simulink model "Integration2022b_May06"  (R2022b)
settings: Solver=FixedStepAuto  StartTime=0.0  StopTime=inf  RelTol=1e-3
model workspace (MAT data in the model file):
  L = 4.165
  SL_ROS_VariableLengthArrays_MaxSizes : object (value not decoded)
  finalint = 0
  firstWarning = 1
  originalScenarioChecksum = '114339432DE22364D47BB28FC96DC10C'
values from neighbouring files (symbols this model uses):
  D = cross(B-A,C-A)    [HelperCalculateEgoRefPathInfo.m]
  data =     [Part_of_MCity.mat]    (also in curvedroad_Bhanu.mat; plotWPScript.m = [data, [out.x.Data(:, :, i); out.y.Data(:, :, i)]])
  x = [Vertices(Na,1) Vertices(:,1) Vertices(Nb,1)]    [HelperCalculateEgoRefPathInfo.m]    (also in HelperConvertDSPoseToSim3D.m = actor(1).Position(1); xpts.mat = [-29.9023190589 -34.2715935353 -19.4160603154 -19.4160603154)
  y = [Vertices(Na,2) Vertices(:,2) Vertices(Nb,2)]    [HelperCalculateEgoRefPathInfo.m]    (also in HelperConvertDSPoseToSim3D.m = actor(1).Position(2); VehicleOutputFcn.m = [x(1);x(2); x(3); x(4); x(5);x(6)]; ypts.mat = [-62.3254015256 -62.9079714558 -51.8391427821 -48.6350081661)
  z = zeros(1, length(interpX))    [HelperCalculateEgoRefPathInfo.m]
undefined symbols (not defined in the file or in its folder): MinVelocity, WB
libraries: ros2lib x13, mpcsigdimcheck_private x10, robotalgslib x1, mpclib x1, drivingvehiclecontroller x1, slpidlib x1
(part 4 of 5)

== matlab function Integration2022b_May06/Environment // SF Detections ==
  data: matrixA input; objectAhead output; mostImpObjectPose output; objectRelativeVelocity output; objectDistance output; railroadGate output; sceneId output; noLight output; red output; yellow output; green output; trafficSignalType output; trafficSignType output; egoLane output; minRelativeVelocity output; minRelativeDistance output; nextRoadSpeed output; roadSpeed output; leftLaneMarkInfo output; rightLaneMarkInfo output; laneNumber output; LatDistanceToScene output; LongDistanceToScene output; matrixB input; matrixC input; matrixD input; matrixE input; matrixF input; transitionFlag input; roadSpeed input; defaultRoadSpeed input; SDist input; CurrentPose input; signX output; signY output
function [objectAhead, mostImpObjectPose, objectRelativeVelocity, objectDistance, railroadGate, sceneId,...
            noLight, red, yellow, green, trafficSignalType, trafficSignType, egoLane, minRelativeVelocity, minRelativeDistance, nextRoadSpeed, roadSpeed, ...
            leftLaneMarkInfo, rightLaneMarkInfo, laneNumber, LatDistanceToScene, LongDistanceToScene, signX, signY] = ...
            PerceptionData(matrixA, matrixB, matrixC, matrixD, matrixE, matrixF, transitionFlag, roadSpeed, ...
            defaultRoadSpeed, SDist, CurrentPose)
 
    % Get sizes of matrices
    sizeA = size(matrixA);                              % Object detections, 
    sizeB = size(matrixB);                              % Traffic signals,
    sizeC = size(matrixC);                              % Traffic signs
    sizeD = size(matrixD);                              % Road state
    sizeE = size(matrixE);                              % Limit line
    sizeF = size(matrixF);                              % Lane markings
    offsetToFront = 2.1336;                             % Offset to the front of the vehicle, from the driver's seat
    % lengthOfCar = 4.1656;                             % Car length
    % Initialization: relevant to matrix A
    objectAhead = 0;                                    % Boolean
    railroadGate = 0;                                   % Boolean
    mostImpObjectPose = zeros(2, 1);
    objectDistance = 40;
    objectRelativeVelocity = 0;                         % [changed from 10 to 0]
    sceneId = 0; 

    % Initialization: relevant to matrix B
    noLight = 0;                                        % Boolean
    trafficSignalType = 0;
    red = zeros(1,6);                                   % Encoded as boolean
    green = zeros(1,3);                                 % Encoded as boolean
    yellow = zeros(1,6);                                % Encoded as boolean
    trafficSignalId = 0;
    % Initialization: relevant to matrix C
    trafficSignType = 0;
    LongDistanceToScene = -1;
    LatDistanceToScene = -1;
    nextRoadSpeed = 7;
    LongDistanceToTrafficSign = 40;
    LatDistanceToTrafficSign=10;
   

    LongDistanceToTrafficSignal = 40;
    LatDistanceToTrafficSignal = 10;
    maxIntersectionLength = 32;                         % Dimension of intersection [m]
    % roadSpeed = defaultRoadSpeed;                       % Initialize to default road speed [mph]
    signLatPose=-1;
    signLongPose=-1;
    egoLane = matrixD(1, 4);
    laneNumber = matrixD(1, 9);
    
    % Relative to ego coordinates
    leftLaneIndex = 0;                                  % Index of left lane marking
    rightLaneIndex = 0;                                 % Index of right lane marking
    leftLaneMarkInfo = zeros(1, 2);                     % Color and type of lane marking
    rightLaneMarkInfo = zeros(1, 2);                    % Color and type of lane marking
    distanceToLaneMarking = zeros(1, sizeF(1));
    
    for i = 1:sizeA(1)                                  % Looping over rows of Matrix A (Different Detections)
       objObjectId = matrixA(i, 1);                     % Object ID
       objObjectType = matrixA(i, 2);                   % Object type
       
       if objObjectType == -1
           break;
       end
    
       lateralPose = matrixA(i, 3);                     % Relative lateral (X) Pose
       longitudinalPose = matrixA(i, 4);                % Relative longitudinal (Y) Pose
       relativeLongVelocity = matrixA(i, 5);            % Relative longitudinal velocity
       relativeLateralVelocity = matrixA(i, 6);         % Relative lateral velocity
       relativeLane = matrixA(i, 7);                    % Relative lane
       dynamicProperty = matrixA(i, 8);                 % Dynamic property (static/dynamic)
       objectCourse = head - (90 - matrixA(i, 9));      % heading in IMU frame (North = 0, clockwise shift) converted to vehicle frame
       netRelativeVelocity = sqrt(relativeLongVelocity^2 + relativeLateralVelocity^2);

    % Static obstacles in our lane
        if (dynamicProperty == 1 && relativeLane == 1) || objObjectId == 5 && (longitudinalPose <= SDist)
            statObstacleFlag = 1;
            statObstacleLocation = double([objectLatitude objectLongitude]);
        end
    % Relative Lane Code = 2: opposing, 3: left lane, 4: right lane 
    % Dynamic obstacles detection
        if (objObjectType > 0 && objObjectType <= 3) && (dynamicProperty == 3 || dynamicProperty == 4) % check if moving vehicle
            if relativeLane == 1 && (objectCourse >= CurrentPose(3) - 15 && objectCourse <= CurrentPose(3) + 15) % cushion of 15 degrees +/- ego vehicle heading to detect same direction travel
                dynamicACCFlag = 1;
                objectAhead = 1;
                objectDistance = min(objectDistance, longitudinalPose); % change to lat/long reading
            end

            if relativeLane == 2 && abs(objectCourse) > 160 && abs(objectCourse < 290) % discuss where relative heading angle starts from: car x or car y or keep it local heading only?
                oppVehicleFlag = 1;

            end
            if relativeLane > 2 && relativeLane < 6 && objectCourse >= 90 - 15 && objectCourse < 90 + 15
                vehicleFlag = 1;
            end

    % Pedestrian at Crosswalk
       if objObjectType == 4 && (relativeLane > 1 && relativeLane < 7) && (dynamicProperty == 3 || dynamicProperty == 4) % check if moving pedestrian (lane, moving, pedestrian check)
           pedestrianFlag = 1;
           objectAhead = 1;
           pedestrianDistance = 
           pedestrianVelocity = netRelativeVelocity;
       end

       if longitudinalPose <= objectDistance
          objectRelativeVelocity = relativeLongVelocity;
          % objectTrackedId = objObjectId;
          mostImpObjectPose(1:2, 1) = [lateralPose; longitudinalPose];
       end

          
       
       % railroad gate detected (closed)
       elseif relativeLane == 1 && objObjectType == 7 
           railroadGate = 1;
       end
end

    
    % Checking which traffic sign is important, its type and position
    for i = 1:sizeC(1)
        % if no detection, scene variables should be -1
%         signLateralPose = matrixC(i, 3);
%         signLongitudinalPose = matrixC(i, 4);
        signObjectId = matrixC(i, 1);
        signType = matrixC(i, 2);
        signX = matrixC(i, 6);
        signY = matrixC(i, 7);
        
        
        % distanceToTrafficSign = sqrt(signX^2 + signY^2);
        if signObjectId == -1 % || matrixD(1, 8) == -1
            break;
        else
            % if there's a known sign and it is not a speed limit
            val1 = (signX - CurrentPose(1))*sind(CurrentPose(3));
            val2 = (signY - CurrentPose(2))*cosd(CurrentPose(3));
            val3 = (signX - CurrentPose(1))*cosd(CurrentPose(3));
            val4 = (signY - CurrentPose(2))*sind(CurrentPose(3));
            signLongitudinalPose = (signX - CurrentPose(1))*sind(90 - CurrentPose(3)) + (signY - CurrentPose(2))*cosd(90 - CurrentPose(3));
            signLateralPose = (signX - CurrentPose(1))*cosd(90 - CurrentPose(3)) - (signY - CurrentPose(2))*sind(90 - CurrentPose(3)); % signY - CurrentPose(2);
            
            if signObjectId > 0 && signType > 2
                LongDistanceToTrafficSign = min(LongDistanceToTrafficSign, abs(signLongitudinalPose));

                % most important traffic sign
                if abs(signLongitudinalPose) <= LongDistanceToTrafficSign
                   trafficSignType = signType;
                   
                   LatDistanceToTrafficSign = signLateralPose;
                   LongDistanceToTrafficSign = signLongitudinalPose;
                end

            elseif signObjectId > 0 && (signType > 0 && signType <= 2)
                
                if signType == 1
                    if (matrixD(1, 2) <= roadSpeed) && matrixD(1, 3) < 8             % set velocity-distance linear equation
                        roadSpeed = matrixD(1, 2);
                        nextRoadSpeed = matrixD(1, 2);
                    elseif matrixD(1, 8) ~= 0
                        roadSpeed = matrixD(1, 8);
                        nextRoadSpeed = matrixD(1, 2);
                    else
                        roadSpeed = defaultRoadSpeed;
                        nextRoadSpeed = matrixD(1, 2);
                    end
%                 elseif signType == 2
%                     if matrixD(1, 8) ~= roadSpeed
%                         roadSpeed = matrixD(1, 8) * 0.621;
%                     else
%                         roadSpeed = roadSpeed;
%                     end
                end              
                
            end
        
        end
    end
    
    % Checking which traffic light is important, its colour and position
    for i = 1:sizeD(1)
        
        % No active traffic light detected
        if matrixD(i, 1) == 0
            break;
        else
            % For all traffic light detections
            for j = 1:sizeB(1)
        
                if matrixB(j, 1) == -1
                    break;
                else
                    trafficSignalId = matrixD(i, 1);
                    signalObjectId = matrixB(j, 1);
                    signalHeadType = matrixB(j, 2);
%                     signalLateralPose = matrixB(j, 3);
%                     signalLongitudinalPose = matrixB(j, 4);
                    signalX = matrixB(j, 21);
                    signalY = matrixB(j, 22);
                    signalLongitudinalPose = (signalX - CurrentPose(1))*cosd(90 - CurrentPose(3)) - (signalY - CurrentPose(2))*sind(90 - CurrentPose(3));
                    signalLateralPose = (signalX - CurrentPose(1))*sind(90 - CurrentPose(3)) + (signalY - CurrentPose(2))*cosd(90 - CurrentPose(3));
            
                    % making sure same traffic light is being referred to
                    if trafficSignalId == signalObjectId
            
                        % [solid, flashing, left, flashingLeft, right, flashingRight]
                        red = [matrixB(j, 6), matrixB(j, 9), matrixB(j, 11), matrixB(j, 14), matrixB(j, 16), matrixB(j, 19)];
                        
                        % [solid, flashing, left, flashingLeft, right, flashingRight]
                        yellow = [matrixB(j, 7), matrixB(j, 10), matrixB(j, 12), matrixB(j, 15), matrixB(j, 17), matrixB(j, 20)];
                        
                        % [1:solid, 2:left, 3:right]
                        green = [matrixB(j, 8), matrixB(j,13), matrixB(j, 18)];
                        
                        noLight = matrixB(j, 5);
                        trafficSignalType = signalHeadType;  
                        LongDistanceToTrafficSignal = signalLongitudinalPose;
                        LatDistanceToTrafficSignal = signalLateralPose;
                    end
                end
            end
        end
    end
    
    %{
        if traffic signal distance is less than traffic sign distance
        distance to the limit line is determined here
    %}
    if LongDistanceToTrafficSignal < LongDistanceToTrafficSign
        sceneId = 8;                    % For a Traffic Light
        LongDistanceToScene = LongDistanceToTrafficSignal;
        LatDistanceToScene = LatDistanceToTrafficSignal;
        
        
        for i = 1:sizeE(1)
            if matrixE(i, 1) == -1
                break;
            else   
%                 limitLineLongitudinalPose = matrixE(i, 3);
%                 limitLineLateralPose = matrixE(i, 2);
                
                limitLineX = matrixE(i, 5); 
                limitLineY = matrixE(i, 6);
                limitLineLongitudinalPose = (limitLineX - CurrentPose(1))*sind(90 - CurrentPose(3)) + (limitLineY - CurrentPose(2))*cosd(90 - CurrentPose(3));
                limitLineLateralPose = (limitLineX - CurrentPose(1))*cosd(90 - CurrentPose(3)) - (limitLineY - CurrentPose(2))*sind(90 - CurrentPose(3)); % limitLineY - CurrentPose(2);

                
%                 relDistanceToLimitLine = norm([limitLineLongitudinalPose,limitLineLateralPose]);
                

%                 limitLineLateralPose = CurrentPose(1) + offsetToFront*cosd(CurrentPose(3)) + relDistanceToLimitLine*cosd(atan2d(limitLineLongitudinalPose,limitLineLateralPose));
%                 limitLineLongitudinalPose = CurrentPose(2) + offsetToFront*sind(CurrentPose(3)) + relDistanceToLimitLine*sind(atan2d(limitLineLongitudinalPose,limitLineLateralPose));
                
                % Below: 
                if matrixE(i, 4) == 1
                    LongDistanceToScene = limitLineLongitudinalPose ;
                    LatDistanceToScene = limitLineLateralPose;
                else
                    if matrixE(i, 1) ~= 0
                        LongDistanceToScene = limitLineLongitudinalPose;
                        LatDistanceToScene = limitLineLateralPose;
                    else
                        LongDistanceToScene = LongDistanceToTrafficSignal - maxIntersectionLength; % modify as of April 28!
                        LatDistanceToScene = LatDistanceToTrafficSignal; % Dummy Value: Modify case above. Lateral Distance is Needed.
                    end
                    
                end
            end
        end
    
    elseif LongDistanceToTrafficSignal > LongDistanceToTrafficSign
        for i = 1:sizeE(1)
            if matrixE(i,1) == -1
                break;
            else
                limitLineX = matrixE(i, 5);
                limitLineY = matrixE(i, 6);
                limitLineLongitudinalPose = (limitLineX - CurrentPose(1))*sind(90 - CurrentPose(3)) + (limitLineY - CurrentPose(2))*cosd(90 - CurrentPose(3));
                limitLineLateralPose = (limitLineX - CurrentPose(1))*cosd(90 - CurrentPose(3)) - (limitLineY - CurrentPose(2))*sind(90 - CurrentPose(3)); % limitLineY - CurrentPose(2);

%                 relDistanceToLimitLine = norm([limitLineLongitudinalPose,limitLineLateralPose]);
%                 limitLineLateralPose = 0*CurrentPose(1) + offsetToFront*cosd(CurrentPose(3)) + relDistanceToLimitLine*cosd(atan2d(limitLineLongitudinalPose,limitLineLateralPose));
%                 limitLineLongitudinalPose = 0*CurrentPose(2) + offsetToFront*sind(CurrentPose(3)) + relDistanceToLimitLine*sind(atan2d(limitLineLongitudinalPose,limitLineLateralPose));
                
                if matrixE(i, 4) == 1
                    LongDistanceToScene = limitLineLongitudinalPose;
                    LatDistanceToScene = limitLineLateralPose;
                else
                    LongDistanceToScene = LongDistanceToTrafficSign;
                    LatDistanceToScene = LatDistanceToTrafficSign;
                end
%                 LongDistanceToScene = LongDistanceToTrafficSign;
%                 LatDistanceToScene = LatDistanceToTrafficSign;
            end
        end
        % LongdistanceToScene = LongdistanceToTrafficSign;   
        % LatDistanceToScene = LatDistanceToTrafficSign;
        switch trafficSignType
            case 3
                sceneId = 7;                % Stop sign
            case 4
                sceneId = 6;                % Yield sign
            case 10
                sceneId = 10;               % Railroad crossing
            case 11
                sceneId = 11;               % Crosswalk
        end
    end

    % *****************************
    % develop logic for unknown detections (all matrices - traffic lights,
    % signs, limit lines, objects, lane markings
    % *****************************

    % If the ego is transitioning from one scene to another
    if transitionFlag == 1
        minRelativeVelocity = objectRelativeVelocity;
        minRelativeDistance = objectDistance;
    else
        minRelativeVelocity = objectRelativeVelocity;
        minRelativeDistance = min(LongDistanceToScene, objectDistance);
    end

    % Lane markings using matrixF
%     for i = 1:sizeF(1)
%         if matrixF(i, 1) == -1
%             break;
%         else
%             distanceToLaneMarking(i) = matrixF(i, 2); % check with perception about the values of this variable
%             [~, laneIndexLeft] = max(distanceToLaneMarking(distanceToLaneMarking < 0));
%             [~, laneIndexRight] = min(distanceToLaneMarking(distanceToLaneMarking > 0));
%             leftLaneMarkInfo = matrixF(laneIndexLeft, 3:4);
%             rightLaneMarkInfo = matrixF(laneIndexRight, 3:4);
%         end
%     end
end

== matlab function Integration2022b_May06/SF Dynamic ==
  data: matrixA input; matrixC input; dynamicRelativeVelocity output; CurrentPose input; distance2Scene input; signX input; signY input; egoVelocity input
function dynamicRelativeVelocity   = TrafficSignAssist(matrixA, matrixC, CurrentPose, distance2Scene, signX, signY, egoVelocity)

offsetToFront = 2.1336;                             % Offset to the front of the vehicle, from the driver's seat
lengthOfCar = 4.1656;                               % Car length
% Initialization: relevant to matrix A
objectAhead = 0;                                    % Boolean
railroadGate = 0;                                   % Boolean
mostImpObjectPose = zeros(2, 1);
objectRelativeDistance = 40;
dynamicRelativeVelocity = 0;                         % [changed from 10 to 0]

maxAccel = 2;
timeAcc = sceneSpeed/maxAccel;
dd = 0.5 * maxAccel * (timeAcc^2);
timeConstantVel = (19 - dd) / SceneSpeed;
totalTime = timeAcc + timeConstantVel;
timeSafe = 1; % Adjusted for other conditions (e,g. weather, road condition ...)
timeOfArrivalThreshold = totalTime + timeSafe;
vehicleClear2GoFlag = 0;

egoSSPriority = 1;
ToAClearance = 1;
ActorHeading = zeros(4,1);
actorExitang = zeros(4,1);

% tempPriority = zeros(numCars+1,1);
d = zeros(10, 5); % distance, velocity, time, location (wrt ego), exit (leaving ints)
Objang = zeros(10, 1);
% priorityTable = zeros(numCars+1, 5);
egoExitang = egoPose(3) - atan2d(midpoint(2)-egoPose(2),midpoint(1)-egoPose(1)); % 0 deg = straight , + = right
egoExitdist = sqrt((midpoint(2)-egoPose(2))^2+(midpoint(1)-egoPose(1))^2);



%%%%%%%%%%%%%%%%%%
intersectionOffset = 15;
timeOfArrival = 1e3;


for i = 1:sizeA(1)                                  % Looping over rows of Matrix A (Different Detections)
   objObjectId = matrixA(i, 1);                     % Object ID
   objObjectType = matrixA(i, 2);                   % Object type
   
   if objObjectType == -1
       break;
   end


   lateralPose = matrixA(i, 3);                     % Relative lateral (X) pose
   longitudinalPose = matrixA(i, 4);                % Relative longitudinal (Y) pose

   relativeLongVelocity = matrixA(i, 5);            % Relative longitudinal velocity
   relativeLateralVelocity = matrixA(i, 6);         % Relative lateral velocity

   relativeLane = matrixA(i, 7);                    % Relative lane
   dynamicProperty = matrixA(i, 8);                 % Dynamic property (static/dynamic)

   objectX = matrixA(i, 10);                        % Object X
   objectY = matrixA(i, 11);                        % Object Y

   objectCourse = matrixA(i, 9));                   % heading in IMU frame converted to vehicle frame

   objectHeading = 90 - objectCourse;
   if objectHeading < -180
       objectHeading = objectHeading + 360;
   elseif abs(objectHeading) == 180
       objectHeading = abs(objectHeading);
   end

   netRelativeVelocity = sqrt(relativeLongVelocity^2 + relativeLateralVelocity^2);


% Relative Lane Code = 2: opposing, 3: left lane, 4: right lane

% Dynamic obstacles detection
    if (objObjectType > 0 && objObjectType <= 3) && (dynamicProperty == 2 || dynamicProperty == 3 && dynamicProperty == 4) % check if moving vehicle
        % First if condition: ACC flag
        if relativeLane == 1 && longitudinalPose <= objectRelativeDistance && (objectCourse >= CurrentPose(3) - 15 && objectCourse <= CurrentPose(3) + 15) % cushion of 15 degrees +/- ego vehicle heading to detect same direction travel
            dynamicACCFlag = 1;
            objectRelativeDistance = longitudinalPose;
            if relativeLongVelocity < 0
                dynamicRelativeVelocity = -netRelativeVelocity;
            else
                dynamicRelativeVelocity = netRelativeVelocity;         % net relative velocity if velocity >= 0
            end
            
        end
        

        % Second if condition: Incoming vehicle (clear 2 go) flag
        offsetAngle = CurrentPose(3) + 45;

        if offsetAngle > 180
            offsetAngle = (offsetAngle - 360);

        intersectionMidpt = [signX + intersectionOffset*cosd(offsetAngle); signY + intersectionOffset*sind(offsetAngle)];
        % incoming vehicles to midpoint

        incomingAngle = atan2d(intersectionMidpt(2) - objectY, intersectionMidpt(1) - objectX);
        objDistanceMidpt = norm(intersectionMidpt - [objectX; objectY]); % distance from incoming ehicle to intersection midpt
        % if objDistanceMidpt > 1e4
        %     objDistanceMidpt = 100;

        velocityXY = [cosd(90 - CurrentPose(3)) -sind(90 - CurrentPose(3)); sind(90 - CurrentPose(3)) cosd(90 - CurrentPose(3))]' * [relativeLateralVelocity; relativeLongVelocity];


        if velocityXY > 0.05
            timeOfArrival = min(timeOfArrival, objDistanceMidpt/velocityXY);
        end
        
        if  ~(abs(incomingAngle) < 45 && objDistanceMidpt <= 30 && timeOfArrival <= timeOfArrivalThreshold) % discuss where relative heading angle starts from: car x or car y or keep it local heading on
            vehicleClear2GoFlag = 1; 
        end

    

        % if relativeLane > 2 && relativeLane < 6 && objectCourse >= 90 - 15 && objectCourse < 90 + 15
        %     vehicleClear2GoFlag = 1;
        % end
    end

    
%%%%%%%%%%%%%%%%%%%%%%%%%%%%%%%%%%%%%%%%%%%%%%%%%%%%%%%%%%%%%%%%%%

% Pedestrian at Crosswalk
   
    if objObjectType == 4 && (relativeLane >= 1 && relativeLane <= 8) && (dynamicProperty == 3 || dynamicProperty == 4) % check if moving pedestrian (lane, moving, pedestrian check)
        relativePedestrianHeading = objectCourse - CurretnPose(3);
        if abs(relativePedestrianHeading)> 180
            relativePedestrianHeading = relativePedestrianHeading - 360;
        elseif abs(relativePedestrianHeading) == 180
            relativePedestrianHeading = abs(relativePedestrianHeading);
        end
        if abs(relativePedestrianHeading) > 45 && abs(relativePedestrianHeading) < 120
            pedestrianFlag = 1;
            pedestrianDistance = 
            pedestrianVelocity = netRelativeVelocity;
    end



      
   
   % % railroad gate detected (closed)
   % elseif relativeLane == 1 && objObjectType == 7 
   %     railroadGate = 1;
   % end
end

== matlab function Integration2022b_May06/StopSignPriority ==
  settings: updateMethod=DISCRETE
  data: ToAClearance output; SDist input; D2S input; ObjTracks input; egoSSPriority output; SceneTracks input; egoPose input; egoSpeed input; numSS output; SceneSpeed input; WB input; d output; flag input; flag output; midpoint input; midpoint output; egoExit output; egoEnter input; egoEnter output; process input; process output
function [ToAClearance, egoSSPriority, numSS, d, flag, midpoint, egoExit, egoEnter, process]  = StopSignPriority(SDist, D2S, ObjTracks, SceneTracks, egoPose, egoSpeed, SceneSpeed, WB, flag, midpoint, egoEnter, process)
% calculate covariance matrix outside, input to this block is modified with final, unique detections
egoPose = [-egoPose(2) egoPose(1) 90+egoPose(3)];
persistent SSPriority C1x C2y C3x C4y
% find stop signs + one of 2way or 4way or T-junction

% find number of signs (until we reach 0 valued columns)
numSS = 0;
for j = 1:length(SceneTracks(1,:))
    if any(SceneTracks(:,j))
        numSS = numSS + 1;
    end
end

% find number of cars
numObjects = 0;
for j = 1:length()
    if any(ObjTracks(:,j))
        numObjects = numObjects + 1;
    end
end


egoSSPriority = 1;
ToAClearance = 1;
ActorHeading = zeros(4,1);
actorExitang = zeros(4,1);
amax = 3;
ta = SceneSpeed/amax;
dd = 0.5*amax*(ta^2);
tcs = (19-dd)/SceneSpeed;
tt = ta + tcs;
tsafe = 1; % Adjusted for other conditions (e,g. weather, road condition ...)
ToAThreshold = tt + tsafe;
% tempPriority = zeros(numCars+1,1);
d = zeros(10, 5); % distance, velocity, time, location (wrt ego), exit (leaving ints)
Objang = zeros(10, 1);
% priorityTable = zeros(numCars+1, 5);
egoExitang = egoPose(3) - atan2d(midpoint(2)-egoPose(2),midpoint(1)-egoPose(1)); % 0 deg = straight , + = right
egoExitdist = sqrt((midpoint(2)-egoPose(2))^2+(midpoint(1)-egoPose(1))^2);

if abs(egoExitang) >= 135 && egoExitdist >= 10
    d(1,5) = 1; % ego left the ints
    egoEnter = 0;
    flag = 0;
elseif abs(egoExitang) >= 135 && egoExitdist <= 20 && egoExitdist >= 10
    d(1,5) = 1;
end

egoExit = d(1,5);


if (D2S <= SDist || egoEnter == 1) && process % && egoExitdist >= 12

    % [~, index] = min(abs(SceneTracks(1,:)'));
    if numSS > 0

        Vmd = [-egoSpeed*sind(egoPose(3)), egoSpeed*cosd(egoPose(3))];
        rot = [cosd(egoPose(3)) -sind(egoPose(3)); sind(egoPose(3)) cosd(egoPose(3))];
        

        % intersection region
        if flag == 0
            C1x = min(SceneTracks(1, 1:numSS)) - (WB + 3);
            C2y = min(SceneTracks(3, 1:numSS)) - (WB + 3);
            C3x = max(SceneTracks(1, 1:numSS)) + (WB + 3);
            C4y = max(SceneTracks(3, 1:numSS)) + (WB + 3);
            C1 = rot*[C1x; C2y] + egoPose(1:2)';
            C2 = rot*[C3x; C4y] + egoPose(1:2)';
            midpoint = (C1+C2)./2;
            
            % C1x = min(SceneTracks(1, 1:numSS)) - (WB + 3);
            % C2y = min(SceneTracks(3, 1:numSS)) - (WB + 3);
            % C3x = max(SceneTracks(1, 1:numSS)) + (WB + 3);
            % C4y = max(SceneTracks(3, 1:numSS)) + (WB + 3);
            % midpoint = [2*egoPose(1)-C4y-C2y; 2*egoPose(2)+C1x+C3x]./2;
        %   scatter(-SceneTracks(3,:)+egoPose(1),SceneTracks(1,:)+egoPose(2),'blue','filled')   
            % scatter(midpoint(1), midpoint(2), 'blue', 'filled')
            % rectangle('Position',[egoPose(1)-C4y egoPose(2)+C1x abs(C4y-C2y) abs(C3x-C1x)])
            flag = C1x;
        end

        midpoint_ego = rot'*(midpoint - egoPose(1:2)');
        
        % loop through num of cars (j)
    
        d(1,1) = sqrt((midpoint(1) - egoPose(1))^2 + (midpoint(2) - egoPose(2))^2);
        d(1,2) = egoSpeed;
        d(1,3) = d(1,1)/d(1,2);     %add ego TOA
        d(1,4) = 4; % 4 is the location of the ego vehicle itself
        
        % if d(1,1) <= 3
        %     ToAThreshold = 2;
        % else
        %     ToAThreshold = 6;
        % end

        if d(1,1) <= flag
            egoEnter = 1;
        end

    
        % loop through signs (vectorized)
        % if smallest dist 
        % d(:,3) -> TOA = v/dist
    
        if numObjects > 0
            for k = 1:numObjects
                d(k+1,1) = sqrt((midpoint_ego(2)-ObjTracks(3,k))^2+(midpoint_ego(1)-ObjTracks(1,k))^2); %sqrt((midpoint(1) - (-ObjTracks(3,k)+egoPose(1)))^2 + (midpoint(2) - (ObjTracks(1,k)+egoPose(2)))^2); 
                d(k+1,2) = sqrt((Vmd(1) - ObjTracks(2,k))^2 + (Vmd(2) - ObjTracks(4,k))^2);
                d(k+1,3) = d(k+1,1)/d(k+1,2); % TOA of other cars
                Objang(k) = atan2d(ObjTracks(1,k), -ObjTracks(3,k));
                                
                % Identify cars location (direction) wrt ego
                if Objang(k) <= 60
                    d(k+1,4) = 1; % 1 = E, 2 = N, 3 = W
                elseif Objang(k) > 60  && Objang(k) < 120
                    d(k+1,4) = 2; % 1 = E, 2 = N, 3 = W
                elseif Objang(k) >= 120
                    d(k+1,4) = 3; % 1 = E, 2 = N, 3 = W
                end

                % Identifying leaving cars
                
                % ActorHeading = atan2d(ObjTracks(2,k) - Vmd(1), -ObjTracks(4,k) - Vmd(2));
                ActorHeading(k) = atan2d(ObjTracks(2,k), ObjTracks(4,k));
                actorExitTheta = ActorHeading(k) - atan2d(midpoint_ego(1)-ObjTracks(1,k),midpoint_ego(2)-ObjTracks(3,k));
                if actorExitTheta > 180
                    actorExitang(k) = actorExitTheta - 360;
                elseif actorExitTheta < -180
                    actorExitang(k) = actorExitTheta + 360;
                else
                    actorExitang(k) = actorExitTheta;
                end
                %actorExitdist = sqrt((midpoint_ego(2)-ObjTracks(3,k))^2+(midpoint_ego(1)-ObjTracks(1,k))^2);
                

                if abs(actorExitang(k)) >= 135 && d(k+1,1) >= 10 
                    d(k+1,5) = 1; % left the ints
                else
                    d(k+1,5) = 0; % did not leave
                end

    
            end
    
            if numSS == 4 
                % Assign priorities based on rank TOA #1, before vehicle stops
                % d1 = d(d(:,1)~=0,:);
                [car, SSPriority] = sort(d(d(:,1)~=0 & d(:,5)==0));
                % priorityTable(:, 1:2) = [car, priority];
        
                tempPriority = find(SSPriority == 1); % ego SS priority
                if ~isempty(tempPriority)
                    egoSSPriority = tempPriority(1);
                end
            
            elseif numSS >= 1 && numSS < 4
                [car, SSPriority] = sort(d((d(:,4)==2 | d(:,4)==4) & d(:,5)==0));
                tempPriority = find(SSPriority == 1); % ego SS priority
                if ~isempty(tempPriority)
                    egoSSPriority = tempPriority(1);              
                end
                ToAClearance = double(all(d(d(:,1)~=0 & d(:,5)==0 & d(:,4)~=4,3) > ToAThreshold));
                
            end
    
        end
    end
    
    
    if ToAClearance == 1 && egoSSPriority == 1 && egoEnter == 1
        process = 0;
    else
        process = 1;
    end
    
    % if egoSpeed <= VelStop
    %     if SSPriority ~= 1
    %         % for all vehicles with higher priority
    %         % provide indicator signals to identify conflicts
    %         % check indicator signs/conflicts and update priority based on that
    %         % code to define leavingScene for other vehicles:
    %         % update priority table
    % 
    %     end
    % end
    
    
    
    

% elseif egoExit == 0
    

end

== stateflow chart Integration2022b_May06/Behavioural Planner/Chart ==
  settings: updateMethod=DISCRETE  sampleTime=0.01
  state Stationary
    en, du:
    desiredVelocity = 0;
    currentDesiredVelocity = desiredVelocity;
    navigate = Navigate;
    transitionFlag = 0;
    timeGap = 1;
    slowDownFlag = 0;
    holdBrake = 1;
  state Navigation
    state Yield [commented out]
      state ApproachingScene [commented out]
        en:
        %brakingFlag = 1;
        transitionFlag = 0;
        timeGap = 0;
      state SlowDown [commented out]
        en, du:
        %desiredVelocity = 0;
        slowDownFlag = 1;
        %ACC = 1; % trying this
        %currentDesiredVelocity = desiredVelocity;
      state Wait [commented out]
        en, du:
        currentDesiredVelocity = desiredVelocity;
        holdBrake = 1;
      state Transition [commented out]
        en, du:
        transitionFlag = 1;
        slowDownFlag = 0;
        holdBrake = 0;
        timeGap = 1;
        desiredVelocity = SceneSpeed;
        currentDesiredVelocity = desiredVelocity;
      state ExitScene [commented out]
        en:
        exitFlag = 1;
      note: Clear2Go will come from Trafiic Sign Assist Function Outside
      (default) -> Navigation.Yield.ApproachingScene [commented out]
      Navigation.Yield.ApproachingScene -> SlowDown [commented out] : [distance2Scene <= SDist]
      SlowDown -> Navigation.Yield.Transition [commented out] : [clearToGo == 1]
      Navigation.Yield.ApproachingScene -> Navigation.Yield.ExitScene [commented out] : [sceneId ~= 7]
      SlowDown -> Navigation.Yield.Wait [commented out] : [egoVelocity <= 0.01]
      Navigation.Yield.Wait -> Navigation.Yield.Transition [commented out] : [clearToGo == 1]
      Navigation.Yield.Transition -> Navigation.Yield.ExitScene [commented out] : [sceneId == 0 && after(3,sec)]
    state RailroadCrossing [commented out]
      state Approaching [commented out]
        en:
        slowDownFlag = 1;
        timeGap = 0;
        transitionFlag = 0;
      state Stop [commented out]
        en:
        desiredVelocity = 0;
        slowDownFlag = 1;
        currentDesiredVelocity = desiredVelocity;
      state Transition [commented out]
        en:
        timeGap = 1;
        transitionFlag = 1;
        slowDownFlag = 0;
        desiredVelocity = SceneSpeed;
        currentDesiredVelocity = desiredVelocity;
      state ExitScene [commented out]
        en:
        exitFlag = 1;
      (default) -> Navigation.RailroadCrossing.Approaching [commented out]
      Navigation.RailroadCrossing.Approaching -> Navigation.RailroadCrossing.Stop [commented out] : [distance2Scene <= SDist && (RRCross == 1 || objectDistance <= TransDist)]
      Navigation.RailroadCrossing.Transition -> Navigation.RailroadCrossing.Approaching [commented out] : [objectDistance <= TransDist]
      Navigation.RailroadCrossing.Approaching -> Navigation.RailroadCrossing.Transition [commented out] : [RRCross == 0 && objectDistance > TransDist && distance2Scene <= SDist]
      Navigation.RailroadCrossing.Approaching -> Navigation.RailroadCrossing.ExitScene [commented out] : [sceneId ~= 10]
      Navigation.RailroadCrossing.Stop -> Navigation.RailroadCrossing.Transition [commented out] : [RRCross == 0 && objectDistance > TransDist]
      Navigation.RailroadCrossing.Transition -> Navigation.RailroadCrossing.ExitScene [commented out] : [sceneId == 0]
    state RoundAbout [commented out]
      state Approaching [commented out]
        en:
        slowDownFlag = 1;
        transitionFlag = 0;
        timeGap = 0;
      state Stop [commented out]
        en:
        desiredVelocity = 0;
        slowDownFlag = 1;
        currentDesiredVelocity = desiredVelocity;
      state ExitScene [commented out]
        en:
        exitFlag = 1;
      state Transition [commented out]
        en:
        timeGap = 1;
        transitionFlag = 1;
        slowDownFlag = 0;
        desiredVelocity = SceneSpeed;
        currentDesiredVelocity = desiredVelocity;
      (default) -> Navigation.RoundAbout.Approaching [commented out]
      Navigation.RoundAbout.Approaching -> Navigation.RoundAbout.Stop [commented out] : [distance2Scene <= SDist]
      Navigation.RoundAbout.Approaching -> Navigation.RoundAbout.ExitScene [commented out] : [sceneId ~= 9]
      Navigation.RoundAbout.Stop -> Navigation.RoundAbout.Transition [commented out] : [clearToGo == 1]
      Navigation.RoundAbout.Transition -> Navigation.RoundAbout.ExitScene [commented out] : [sceneId == 0]
    state destinationCheck
      en,du:
      (default) -> (junction 47)
      (junction 47) -> (junction 48) [order 1] : [distanceToDestination < 2]
      (junction 47) -> (junction 49) [order 2] : {destinationReached = 0;}
      (junction 48) -> (junction 50) : {destinationReached = 1;}
      (junction 50) -> (junction 49)
      (junction 49) -> (junction 51)
    state sceneRecognition
      en,du:
      holdBrake = 0;
      desiredVelocity = roadSpeed;
      currentDesiredVelocity= desiredVelocity;
      exitFlag = 0;
      % Calculate Sdist and curvature slowdown dist here
    state Go
      en:
      desiredVelocity = roadSpeed;
      currentDesiredVelocity = desiredVelocity;
      transitionFlag = 0;
      exitFlag = 0;
    state TrafficLight [commented out]
      note: Yellow light duration is 1s
      state Stop [commented out]
        en, du:
        slowDownFlag = 1;
        desiredVelocity = 0;
        currentDesiredVelocity = desiredVelocity;
      state Approaching [commented out]
        en:
        timeGap = 0;
        transitionFlag = 0;
        T2S = 0;
        slowDownFlag = 1;
      state DecisionOnYellow [commented out]
        en:
        T2S = distance2Scene/egoVelocity;
      state Transition [commented out]
        en, du:
        transitionFlag = 1;
        slowDownFlag = 0;
        timeGap = 1;
        desiredVelocity = SceneSpeed;
        currentDesiredVelocity = desiredVelocity;
      state ExitScene [commented out]
        en:
        exitFlag = 1;
      DecisionOnYellow -> Navigation.TrafficLight.Approaching [commented out] : [T2S > 1.2]
      (default) -> Navigation.TrafficLight.Approaching [commented out]
      Navigation.TrafficLight.Approaching -> Navigation.TrafficLight.Stop [commented out] : [distance2Scene <= SDist]
      Navigation.TrafficLight.Stop -> Navigation.TrafficLight.Transition [commented out] : [greenLight == 1 && objectDistance > TransDist]
      Navigation.TrafficLight.Transition -> Navigation.TrafficLight.Approaching [commented out] : [redLight == 1  || objectDistance < TransDist]
      Navigation.TrafficLight.Approaching -> Navigation.TrafficLight.Transition [commented out] : [greenLight == 1 && objectDistance > TransDist]
      Navigation.TrafficLight.Approaching -> Navigation.TrafficLight.ExitScene [commented out] : [sceneId ~= 8]
      DecisionOnYellow -> Navigation.TrafficLight.Transition [commented out] : [T2S <= 1.2]
      Navigation.TrafficLight.Transition -> DecisionOnYellow [commented out] : [yellowLight == 1]
      Navigation.TrafficLight.Transition -> Navigation.TrafficLight.ExitScene [commented out] : [sceneId == 0]
    state StopSign
      state ApproachingScene
        en:
        transitionFlag = 0;
        timeGap = 0;
      state Stop
        en, du:
        desiredVelocity = 0;
        slowDownFlag = 1;
        %ACC = 1; % trying this
        currentDesiredVelocity = desiredVelocity;
      state Wait
        en, du:
        currentDesiredVelocity = desiredVelocity;
        holdBrake = 1;
      note: To do: Midpoint calculation at Intersection for Transition state behavior
      state ExitScene
        en:
        exitFlag = 1;
      state Transition
        en, du:
        transitionFlag = 1;
        slowDownFlag = 0;
        holdBrake = 0;
        timeGap = 1;
        desiredVelocity = SceneSpeed;
        currentDesiredVelocity = desiredVelocity;
      (default) -> Navigation.StopSign.ApproachingScene
      Navigation.StopSign.ApproachingScene -> Navigation.StopSign.Stop [order 1] : [distance2Scene <= SDist]
      Navigation.StopSign.ApproachingScene -> Navigation.StopSign.ExitScene [order 2] : [sceneId ~= 7]
      Navigation.StopSign.Stop -> Navigation.StopSign.Wait : [egoVelocity <= 0.01  ]
      Navigation.StopSign.Wait -> Navigation.StopSign.Transition : [after(5,sec) && clearToGo == 1]
      Navigation.StopSign.Transition -> Navigation.StopSign.ExitScene : [sceneId == 0 && after(3,sec)]
    state StopSignDyn
      state ApproachingScene
        en:
        transitionFlag = 0;
        timeGap = 0;
      state Stop
        en, du:
        desiredVelocity = 0;
        slowDownFlag = 1;
        %ACC = 1; % trying this
        currentDesiredVelocity = desiredVelocity;
      state Wait
        en, du:
        currentDesiredVelocity = desiredVelocity;
        holdBrake = 1;
      note: To do: Midpoint calculation at Intersection for Transition state behavior
      state ExitScene
        en:
        exitFlag = 1;
      state Transition
        en, du:
        transitionFlag = 1;
        slowDownFlag = 0;
        holdBrake = 0;
        timeGap = 1;
        desiredVelocity = SceneSpeed;
        currentDesiredVelocity = desiredVelocity;
      (default) -> Navigation.StopSignDyn.ApproachingScene
      Navigation.StopSignDyn.ApproachingScene -> Navigation.StopSignDyn.Stop [order 1] : [distance2Scene <= SDist]
      Navigation.StopSignDyn.ApproachingScene -> Navigation.StopSignDyn.ExitScene [order 2] : [sceneId ~= 7]
      Navigation.StopSignDyn.Stop -> Navigation.StopSignDyn.Wait : [egoVelocity <= 0.01  ]
      Navigation.StopSignDyn.Wait -> Navigation.StopSignDyn.Transition : [after(5,sec) && clearToGo == 1]
      Navigation.StopSignDyn.Transition -> Navigation.StopSignDyn.ExitScene : [sceneId == 0 && after(3,sec)]
    Go -> Yield [commented out] : [sceneId == 6]
    sceneRecognition -> Yield [commented out] : [sceneId == 6]
    Yield -> Go [commented out] : [exitFlag == 1]
    Go -> RailroadCrossing [commented out] : [sceneId == 10]
    sceneRecognition -> RailroadCrossing [commented out] : [sceneId == 10]
    RailroadCrossing -> Go [commented out] : [exitFlag == 1]
    Go -> RoundAbout [commented out] : [sceneId == 9]
    (default) -> destinationCheck
    sceneRecognition -> RoundAbout [commented out] : [sceneId == 9]
    RoundAbout -> Go [commented out] : [exitFlag == 1]
    destinationCheck -> sceneRecognition : [destinationReached == 0]
    sceneRecognition -> destinationCheck [order 2] : [distanceToDestination < 2]
    Go -> TrafficLight [commented out] : [sceneId == 8]
    sceneRecognition -> TrafficLight [commented out] : [sceneId == 8]
    TrafficLight -> Go [commented out] : [exitFlag == 1]
    StopSign -> Go : [exitFlag == 1]
    sceneRecognition -> StopSign [order 1] : [sceneId == 7]
    Go -> destinationCheck [order 1] : [sceneId == 0]
    Go -> StopSign [order 2] : [sceneId == 7]
  (default) -> Stationary
  Stationary -> Navigation : [navigate == 1]
  Navigation -> Stationary : [navigate == 0 || destinationReached == 1]
  data: greenLight input; yellowLight input; redLight input; TransDist input; egoVelocity input; objectDistance input; SceneSpeed input; SDist input; RRCross input; distance2Scene input; destinationReached local; exitFlag local; distanceToDestination input; clearToGo input; roadSpeed input; currentDesiredVelocity local; desiredVelocity output double; sceneId input; timeGap output; transitionFlag output; slowDownFlag output; T2S local; Navigate input; navigate local; holdBrake output

== matlab function Integration2022b_May06/Perception Pre-Processing/Subsystem/Curvature ==
  data: RefPose input; CurvatureAhd output; SlowDist input; CurveMinThreshold input
function CurvatureAhd = CurveCalc(RefPose,SlowDist,CurveMinThreshold)

DX = gradient(RefPose(:,1));
D2X = gradient(DX);
DY = gradient(RefPose(:,2));
D2Y = gradient(DY);
curvature = (DX.*D2Y - DY.*D2X) ./(DX.^2+DY.^2).^(3/2);

% calculate distance vector
distancematrix = squareform(pdist(RefPose));
distancesteps = zeros(length(RefPose)-1,1);
for i = 2:length(RefPose)
    distancesteps(i-1,1) = distancematrix(i,i-1);
end
totalDistance = sum(distancesteps); % Total distance travelled [ x y C ] 200x4
distbp = cumsum([0; distancesteps]); % Distance for each waypoint


% r = 1./abs(curvature);
% VelProfile = min(9,sqrt(9.81*r.*0.4*0.9));
st = 0;
en = 1;
j1 = 1;
CurveInfo = zeros(length(curvature),7); % [startX startY endX endY MaxCurve startidx endidx]

for j = 1:length(curvature)
    if abs(curvature(j)) >= CurveMinThreshold
        if abs(curvature(j)) >= CurveInfo(j1,5)
            CurveInfo(j1,5) = abs(curvature(j));
        end
        if st == 0
            CurveInfo(j1,1:2) = [RefPose(j,1) RefPose(j,2)]; % Startpoint
            CurveInfo(j1,6) = j;
            st = 1;
            en = 0;
        end
    elseif (abs(curvature(j)) < CurveMinThreshold) && (en == 0)
            CurveInfo(j1,3:4) = [RefPose(j,1) RefPose(j,2)]; % Endpoint
            CurveInfo(j1,7) = j;
            j1 = j1+1;
            st = 0;
            en = 1;
    end
    if (j == length(curvature)) && (en == 0)
           CurveInfo(j1,3:4) = [RefPose(j,1) RefPose(j,2)]; % Endpoint
            CurveInfo(j1,7) = j;
            j1 = j1+1;
            st = 0;
            en = 1;
    end
end
j2 = 1;
CurvatureAhd = zeros(length(curvature),1);
if j1 > 1
    for j = 1:length(distbp)
        if (distbp(j) >= (distbp(CurveInfo(j2, 6)) - SlowDist)) && (distbp(j) < distbp(CurveInfo(j2,7)))
            CurvatureAhd(j) = CurveInfo(j2,5);
        elseif (distbp(j) >= distbp(CurveInfo(j2,7))) && (j2 < j1-1)
            CurvatureAhd(j) = CurveInfo(j2,5);
            j2 = j2+1;
        else
            CurvatureAhd(j) = curvature(j);
        end
    end
end
